simulink model "Quarter_Suspension_model_with_Sky_Control"  (R2023b)
settings: Solver=ode45  StartTime=0.0  StopTime=10  RelTol=1e-3
values from neighbouring files (symbols this model uses):
  cs = 1000    [Plots_passive.m]
  ct = 50    [Plots_passive.m]
  ks = 15000    [Plots_passive.m]
  kt = 200000    [Plots_passive.m]
  ms = 300    [Plots_passive.m]
  mu = 40    [Plots_passive.m]
undefined symbols (not defined in the file or in its folder): c_sky
settings Model: Creator=DELL  LastModifiedBy=DELL

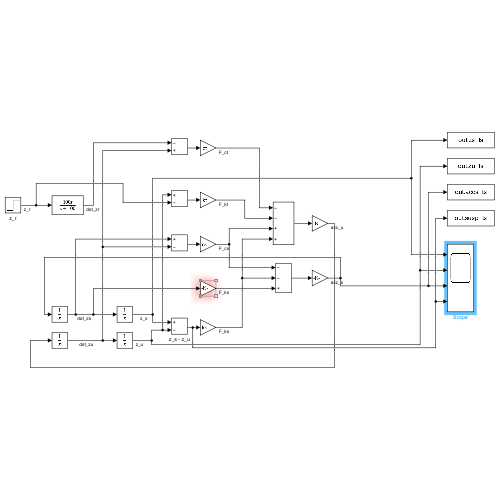
[thumbnail: Simulink's stored preview of the top-level diagram]
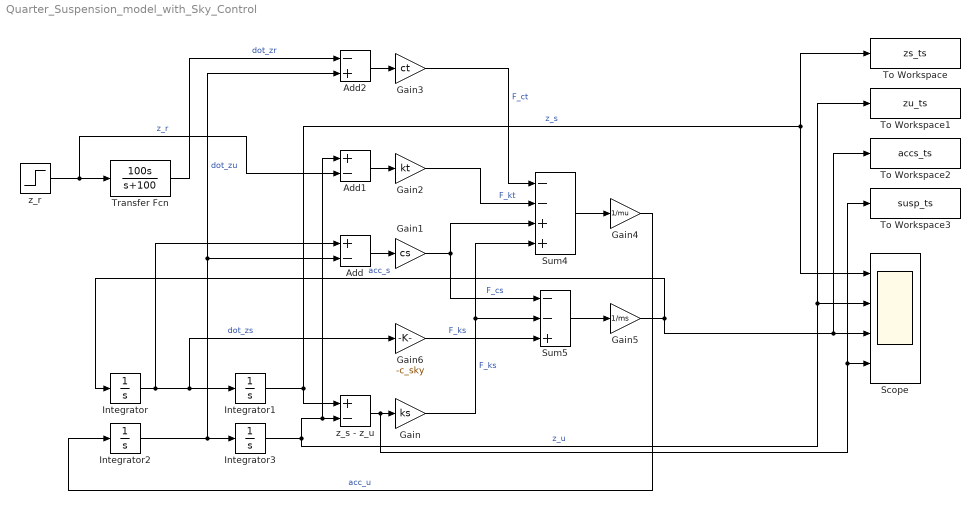
== system Quarter_Suspension_model_with_Sky_Control ==
  Add : Sum  Inputs=+-
  Add1 : Sum  Inputs=+-
  Add2 : Sum  Inputs=-+
  Gain : Gain  Gain=ks
  Gain1 : Gain  Gain=cs
  Gain2 : Gain  Gain=kt
  Gain3 : Gain  Gain=ct
  Gain4 : Gain  Gain=1/mu
  Gain5 : Gain  Gain=1/ms
  Gain6 : Gain  Gain=-c_sky
  Integrator{,1..3} (4 alike) : Integrator
  Scope : Scope  NumInputPorts=4
  Sum4 : Sum  Inputs=--++
  Sum5 : Sum  Inputs=--+
  To Workspace : ToWorkspace  VariableName=zs_ts  SaveFormat=Timeseries  SampleTime=-1
  To Workspace1 : ToWorkspace  VariableName=zu_ts  SaveFormat=Timeseries  SampleTime=-1
  To Workspace2 : ToWorkspace  VariableName=accs_ts  SaveFormat=Timeseries  SampleTime=-1
  To Workspace3 : ToWorkspace  VariableName=susp_ts  SaveFormat=Timeseries  SampleTime=-1
  Transfer Fcn : TransferFcn  Numerator=[100 0]  Denominator=[1 100]
  z_r : Step  After=0.01  SampleTime=0
  z_s - z_u : Sum  Inputs=+-
  wires:
  z_r/1 -> Add1/2, Transfer Fcn/1  "z_r"
  Integrator/1 -> Add/1, Gain6/1, Integrator1/1  "dot_zs"
  Integrator1/1 -> To Workspace/1, Scope/1, z_s - z_u/1  "z_s"
  Integrator2/1 -> Add2/2, Add/2, Integrator3/1  "dot_zu"
  Integrator3/1 -> To Workspace1/1, Scope/2, Add1/1, z_s - z_u/2  "z_u"
  z_s - z_u/1 -> To Workspace3/1, Scope/4, Gain/1
  Add/1 -> Gain1/1
  Add1/1 -> Gain2/1
  Transfer Fcn/1 -> Add2/1  "dot_zr"
  Add2/1 -> Gain3/1
  Gain/1 -> Sum5/2, Sum4/4  "F_ks"
  Gain1/1 -> Sum4/3, Sum5/1  "F_cs"
  Gain2/1 -> Sum4/2  "F_kt"
  Gain3/1 -> Sum4/1  "F_ct"
  Sum4/1 -> Gain4/1
  Gain4/1 -> Integrator2/1  "acc_u"
  Sum5/1 -> Gain5/1
  Gain5/1 -> Integrator/1, To Workspace2/1, Scope/3  "acc_s"
  Gain6/1 -> Sum5/3  "F_ks"
